simulink subsystem "pe2019"  (R2019b)
settings: Solver=VariableStepAuto  StartTime=0.0  StopTime=10.0  RelTol=1e-3
undefined symbols (not defined in the file): chao, smiData, X, Y, Z
libraries: nesl_utility x12, sm_lib x8, Contact_Forces_Lib x4
settings Model: Creator=Franciele Sembay  LastModifiedBy=Franciele Sembay
settings DebuggingCC: UnconnectedInputMsg=none  UnconnectedOutputMsg=none  UnconnectedLineMsg=none  SFMachineParentedDataDiag=error

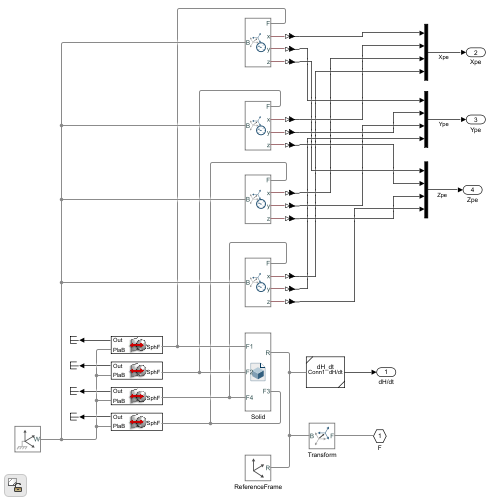
[thumbnail: Simulink's stored preview of the top-level diagram]
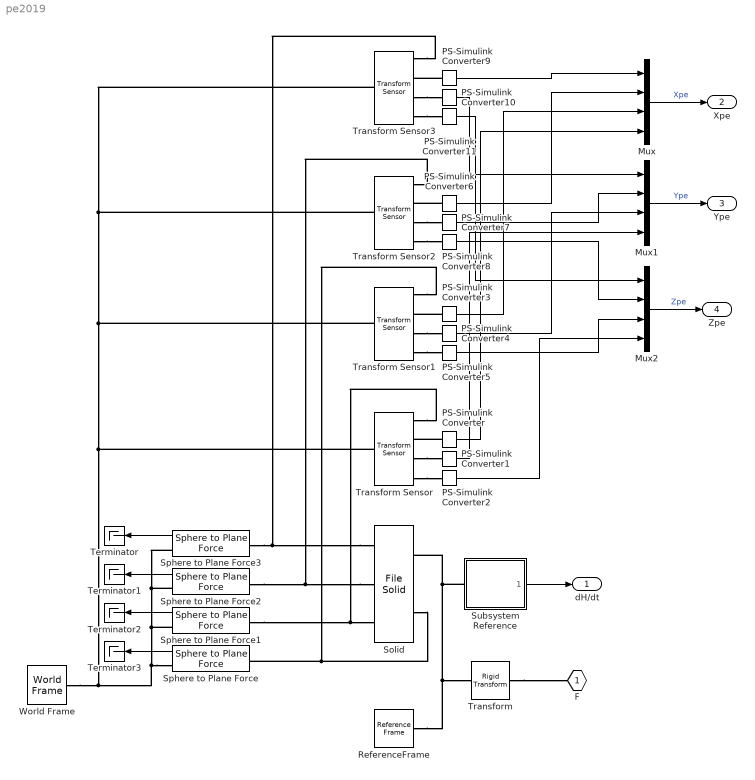
== system pe2019 ==
  Mux : Mux
  Mux1 : Mux
  Mux2 : Mux
  PS-Simulink Converter{,1..11} (12 alike) : nesl_utility/PS-Simulink Converter  PhysicalDomain=network_engine_domain  SubClassName=ps_output  LeftPortType=input  RightPortType=output  PseudoPeriodic=off  Frequencies=[]  VectorFormat=inherit  Unit=inherit  AffineConversion=off
      settings: SourceProductBaseCode=SS,PW,VE
  ReferenceFrame : sm_lib/Frames and Transforms/Reference Frame
  Solid : sm_lib/Body Elements/File Solid  ExtGeomFileName=pe_Valor predeterminado_sldprt.STEP  UnitType=FromFile  ExtGeomFileUnits=m  StepReaderType=HEX  ExportConvexHullGeometry=off  InertiaType=Custom  Mass=smiData.Solid(7).mass  MassUnits=kg  CenterOfMass=smiData.Solid(7).CoM  CenterOfMassUnits=mm  MomentsOfInertia=smiData.Solid(7).MoI  MomentsOfInertiaUnits=kg*mm^2  ProductsOfInertia=smiData.Solid(7).PoI  ProductsOfInertiaUnits=kg*mm^2  BasedOnType=DensityFromFile  Density=1000  DensityUnits=kg/m^3  DoExposeReferenceFrame=on  SerializedFrames=<Frames><Frame><Id>Frame1</Id><Value><Name>F1</Name><Origin><Source>GeometricFeature</Source><FeatureName>point 271</FeatureName></Origin><PrimaryAxis><DefinedDirection>+Z</DefinedDirection><Source>ReferenceFrame</Source><SourceDirection>+Z</SourceDirection><FeatureName></FeatureName></PrimaryAxis><SecondaryAxis><DefinedDirection>+X</DefinedDirection><Source>ReferenceFrame</Source><SourceDirection>+X</SourceDirection><FeatureName></FeatureName></SecondaryAxis></Value></Frame><Frame><Id>Frame2</Id><Value><Name>F2</Name><Origin><Source>GeometricFeature</Source><FeatureName>point 259</FeatureName></Origin><PrimaryAxis><DefinedDirection>+Z</DefinedDirection><Source>ReferenceFrame</Source><SourceDirection>+Z</SourceDirection><FeatureName></FeatureName></PrimaryAxis><SecondaryAxis><DefinedDirection>+X</DefinedDirection><Source>ReferenceFrame</Source><SourceDirection>+X</SourceDirection><FeatureName></FeatureName></SecondaryAxis></Value></Frame><Frame><Id>Frame3</Id><Value><Name>F3</Name><Origin><Source>GeometricFeature</Source><FeatureName>point 269</FeatureName></Origin><PrimaryAxis><DefinedDirection>+Z</DefinedDirection><Source>ReferenceFrame</Source><SourceDirection>+Z</SourceDirection><FeatureName></FeatureName></PrimaryAxis><SecondaryAxis><DefinedDirection>+X</DefinedDirection><Source>ReferenceFrame</Source><SourceDirection>+X</SourceDirection><FeatureName></FeatureName></SecondaryAxis></Value></Frame><Frame><Id>Frame4</Id><Value><Name>F4</Name><Origin><Source>GeometricFeature</Source><FeatureName>point 255</FeatureName></Origin><PrimaryAxis><DefinedDirection>+Z</DefinedDirection><Source>ReferenceFrame</Source><SourceDirection>+Z</SourceDirection><FeatureName></FeatureName></PrimaryAxis><SecondaryAxis><DefinedDirection>+X</DefinedDirection><Source>ReferenceFrame</Source><SourceDirection>+X</SourceDirection><FeatureName></FeatureName></SecondaryAxis></Value></Frame></Frames>  GraphicType=FromGeometry  MarkerShape=Sphere  MarkerSize=10  GraphicVisPropType=SimpleVisualProperties  GraphicDiffuseColor=smiData.Solid(7).color  GraphicSpecularColor=[0.5 0.5 0.5 1.0]  GraphicAmbientColor=[0.15 0.15 0.15 1.0]  GraphicEmissiveColor=[0.0 0.0 0.0 1.0]  GraphicShininess=75  GraphicOpacity=smiData.Solid(7).opacity
  Sphere to Plane Force{,1..3} (4 alike) : Contact_Forces_Lib/3D/Sphere to Plane Force  sphere_rad=SphereRadius  plane_lenx=chao(1)  plane_leny=chao(2)  plane_depth=chao(3)/2  force_law=Linear  k_contact=ContactStiffness  b_contact=ContactDamping  pen_full_damp_F=1e-4  pen_exponent=1  custom_param_1=1  custom_param_2=1  friction_law=Stick-Slip Continuous  mu_kinetic=KinectFriction  mu_static=StaticFriction  v_thr=VelocityThreshold  vis_on=off  vis_opc_en=0  vis_len_plaBz=0.005  vis_clr=[0.9 0.2 0.2]  vis_opc=0.7
  Subsystem Reference : Subsystem  ReferencedSubsystem=dH_dt
  Terminator{,1..3} (4 alike) : Terminator
  Transform : sm_lib/Frames and Transforms/Rigid Transform  TranslationMethod=Cartesian  TranslationStandardOffset=0  TranslationLengthUnit=mm  TranslationStandardAxis=+Z  TranslationCartesianOffset=smiData.RigidTransform(4).translation  TranslationROffset=0  TranslationROffsetUnits=m  TranslationZOffset=0  TranslationZOffsetUnits=m  TranslationThetaOffset=0  TranslationThetaOffsetUnits=deg  RotationMethod=ArbitraryAxis  RotationAngleUnits=rad  RotationStandardAxis=+Z  RotationAngle=smiData.RigidTransform(4).angle  RotationArbitraryAxis=smiData.RigidTransform(4).axis  FollAlignAxisA=+X  BaseAlignAxisA=+Y  FollAlignAxisB=+Y  BaseAlignAxisB=+Z  RotationSequenceAxes=FollowerAxes  RotationSequence=XYX  RotationSequenceAngles=[0 0 0]  RotationSequenceAnglesUnits=deg  RotationMatrix=[1 0 0; 0 1 0; 0 0 1]
  Transform Sensor{,1..3} (4 alike) : sm_lib/Frames and Transforms/Transform Sensor  MeasurementFrame=World  SenseAngle=off  SenseAxis=off  SenseAngle1=off  SenseAngle2=off  SenseAngle3=off  SenseQ=off  SenseR=off  SenseOmegaX=off  SenseOmegaY=off  SenseOmegaZ=off  SenseOmega1=off  SenseOmega2=off  SenseOmega3=off  SenseQDot=off  SenseRDot=off  SenseAlphaX=off  SenseAlphaY=off  SenseAlphaZ=off  SenseAlpha1=off  SenseAlpha2=off  SenseAlpha3=off  SenseQDDot=off  SenseRDDot=off  SenseX=on  SenseY=on  SenseZ=on  SenseRad=off  SenseAzim=off  SenseDist=off  SenseInc=off  SenseXDot=off  SenseYDot=off  SenseZDot=off  SenseRadDot=off  SenseAzimDot=off  SenseDistDot=off  SenseIncDot=off  SenseXDDot=off  SenseYDDot=off  SenseZDDot=off  SenseRadDDot=off  SenseAzimDDot=off  SenseDistDDot=off  SenseIncDDot=off
  World Frame : sm_lib/Frames and Transforms/World Frame
  F : PMIOPort  Side=Left
  dH/dt : Outport
  Xpe : Outport  Port=2
  Ype : Outport  Port=3
  Zpe : Outport  Port=4
  wires:
  Sphere to Plane Force3/1 -> Terminator/1
  Sphere to Plane Force/1 -> Terminator3/1
  Sphere to Plane Force1/1 -> Terminator2/1
  Sphere to Plane Force2/1 -> Terminator1/1
  Subsystem Reference/1 -> dH/dt/1
  PS-Simulink Converter9/1 -> Mux/1
  PS-Simulink Converter6/1 -> Mux/2
  PS-Simulink Converter3/1 -> Mux/3
  PS-Simulink Converter/1 -> Mux/4
  PS-Simulink Converter10/1 -> Mux1/1
  PS-Simulink Converter7/1 -> Mux1/2
  PS-Simulink Converter4/1 -> Mux1/3
  PS-Simulink Converter1/1 -> Mux1/4
  PS-Simulink Converter11/1 -> Mux2/1
  PS-Simulink Converter8/1 -> Mux2/2
  PS-Simulink Converter5/1 -> Mux2/3
  PS-Simulink Converter2/1 -> Mux2/4
  Mux/1 -> Xpe/1  "Xpe"
  Mux1/1 -> Ype/1  "Ype"
  Mux2/1 -> Zpe/1  "Zpe"
  connections:
  ReferenceFrame/RConn1 -- Transform/LConn1 -- Solid/RConn1 -- Subsystem Reference/LConn1
  Sphere to Plane Force/RConn1 -- Sphere to Plane Force3/RConn1 -- Sphere to Plane Force2/RConn1 -- Sphere to Plane Force1/RConn1 -- World Frame/RConn1 -- Transform Sensor/LConn1 -- Transform Sensor1/LConn1 -- Transform Sensor2/LConn1 -- Transform Sensor3/LConn1
  Transform Sensor1/RConn1 -- Solid/RConn2 -- Sphere to Plane Force/LConn1
  Transform Sensor/RConn1 -- Sphere to Plane Force1/LConn1 -- Solid/LConn3
  Solid/LConn1 -- Sphere to Plane Force3/LConn1 -- Transform Sensor3/RConn1
  Solid/LConn2 -- Sphere to Plane Force2/LConn1 -- Transform Sensor2/RConn1
  Transform/RConn1 -- F/RConn1
  PS-Simulink Converter/LConn1 -- Transform Sensor/RConn2
  Transform Sensor/RConn3 -- PS-Simulink Converter1/LConn1
  Transform Sensor/RConn4 -- PS-Simulink Converter2/LConn1
  PS-Simulink Converter3/LConn1 -- Transform Sensor1/RConn2
  Transform Sensor1/RConn3 -- PS-Simulink Converter4/LConn1
  Transform Sensor1/RConn4 -- PS-Simulink Converter5/LConn1
  Transform Sensor3/RConn4 -- PS-Simulink Converter11/LConn1
  PS-Simulink Converter6/LConn1 -- Transform Sensor2/RConn2
  Transform Sensor2/RConn3 -- PS-Simulink Converter7/LConn1
  Transform Sensor2/RConn4 -- PS-Simulink Converter8/LConn1
  PS-Simulink Converter9/LConn1 -- Transform Sensor3/RConn2
  Transform Sensor3/RConn3 -- PS-Simulink Converter10/LConn1
